simulink model "chaodianRM"  (R2021b)
settings: Solver=ode45  StartTime=0.0  StopTime=2  RelTol=1e-3  EnableMultiTasking=on
libraries: spsSeriesRLCBranchLib x9, spsCurrentMeasurementLib x4, spsMeanLib x2, simulink x2, spsVoltageMeasurementLib x2, spsDCVoltageSourceLib x1, spsMosfetLib x1, spsUniversalBridgeLib x1, spspowerguiLib x1
settings Model: SimulationMode=accelerator  Creator=bzz  LastModifiedBy=abc6820292
settings SolverCC: ZeroCrossAlgorithm=Adaptive  AlgebraicLoopSolver=TrustRegion
settings DataIOCC: LimitDataPoints=on  ReturnWorkspaceOutputs=off
settings OptimizationCC: LifeSpan=inf
settings DebuggingCC: AlgebraicLoopMsg=none  IgnoredZcDiagnostic=none  AllowSymbolicDim=off  SFUnexpectedBacktrackingDiag=warning  SFNoUnconditionalDefaultTransitionDiag=warning  SFMachineParentedDataDiag=warning  ArithmeticOperatorsInVariantConditions=warning
settings ModelReferenceCC: PropagateSignalLabelsOutOfModel=off
settings SFSimCC: SimUseLocalCustomCode=off  CustomCodeUndefinedFunction=UseInterfaceOnly
settings RTWCC: RTWUseLocalCustomCode=off
settings CodeAppCC: StateflowObjectComments=on
settings GRTTargetCC: TargetLangStandard=C89/C90 (ANSI)
settings ConfigComp: CovMetricSettings=dw  CovSaveCumulativeToWorkspaceVar=on  CovSaveSingleToWorkspaceVar=on  CovExternalEMLEnable=off
settings SimscapeCC: SimscapeNormalizeSystem=off

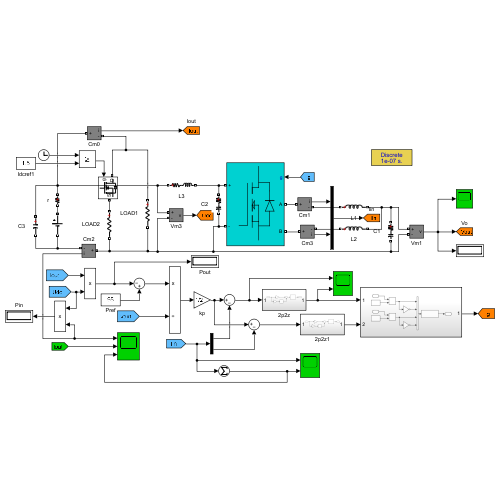
[thumbnail: Simulink's stored preview of the top-level diagram]
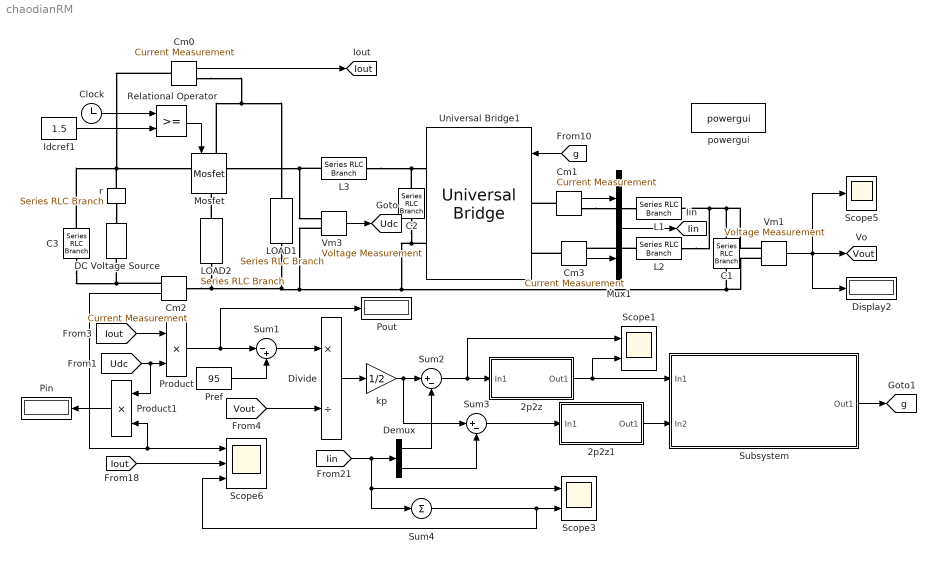
== system chaodianRM ==
  2p2z : Subsystem
  2p2z1 : Subsystem
  C1 : spsSeriesRLCBranchLib/Series RLC Branch  LConnTagsString=__new0  RConnTagsString=__new0  BranchType=RC  Resistance=0.05  Inductance=0  SetiL0=off  InitialCurrent=0  Capacitance=3.33  Setx0=on  InitialVoltage=20  Measurements=None
  C2 : spsSeriesRLCBranchLib/Series RLC Branch  LConnTagsString=__new0  RConnTagsString=__new0  BranchType=RC  Resistance=0.01  Inductance=0  SetiL0=off  InitialCurrent=0  Capacitance=10e-6  Setx0=on  InitialVoltage=24  Measurements=None
  C3 : spsSeriesRLCBranchLib/Series RLC Branch  LConnTagsString=__new0  RConnTagsString=__new0  BranchType=C  Resistance=0.01  Inductance=0  SetiL0=off  InitialCurrent=0  Capacitance=1e-3  Setx0=on  InitialVoltage=24  Measurements=None
  Clock : Clock
  Cm{0..3} (4 alike) : spsCurrentMeasurementLib/Current Measurement  PhasorSimulation=off  OutputType=Complex  PSBequivalent=0
  DC Voltage Source : spsDCVoltageSourceLib/DC Voltage Source  Amplitude=24  Measurements=None
  Demux : Demux  Outputs=2
  Display2 : Display
  Divide : Product  Inputs=*/
  Idcref1 : Constant  Value=1.5
  L1 : spsSeriesRLCBranchLib/Series RLC Branch  LConnTagsString=__new0  RConnTagsString=__new0  BranchType=L  Resistance=0  Inductance=2e-4  SetiL0=off  InitialCurrent=0  Capacitance=inf  Setx0=off  InitialVoltage=0  Measurements=None
  L2 : spsSeriesRLCBranchLib/Series RLC Branch  LConnTagsString=__new0  RConnTagsString=__new0  BranchType=L  Resistance=0  Inductance=2e-4  SetiL0=off  InitialCurrent=0  Capacitance=inf  Setx0=off  InitialVoltage=0  Measurements=None
  L3 : spsSeriesRLCBranchLib/Series RLC Branch  LConnTagsString=__new0  RConnTagsString=__new0  BranchType=RL  Resistance=0.05  Inductance=1e-5  SetiL0=off  InitialCurrent=0  Capacitance=inf  Setx0=off  InitialVoltage=0  Measurements=None
  LOAD1 : spsSeriesRLCBranchLib/Series RLC Branch  LConnTagsString=__new0  RConnTagsString=__new0  BranchType=R  Resistance=24  Inductance=2e-3  SetiL0=off  InitialCurrent=0  Capacitance=inf  Setx0=off  InitialVoltage=0  Measurements=None
  LOAD2 : spsSeriesRLCBranchLib/Series RLC Branch  LConnTagsString=__new0  RConnTagsString=__new0  BranchType=R  Resistance=6  Inductance=2e-3  SetiL0=off  InitialCurrent=0  Capacitance=inf  Setx0=off  InitialVoltage=0  Measurements=None
  Mosfet : spsMosfetLib/Mosfet  Ron=0.1  Lon=0  Rd=0.01  Vfd=0  IC=0  Rs=1e5  Cs=inf  Measurements=off
  Mux1 : Mux  Inputs=2
  Pin : Display
  Pout : Display
  Pref : Constant  Value=95
  Product : Product
  Product1 : Product
  Relational Operator : RelationalOperator  OutDataTypeStr=boolean  RndMeth=Nearest
  Scope1 : Scope  NumInputPorts=2
  Scope3 : Scope  NumInputPorts=2
  Scope5 : Scope
  Scope6 : Scope  NumInputPorts=3
  Subsystem : Subsystem
  Sum1 : Sum  Inputs=|-+
  Sum2 : Sum  Inputs=|+-
  Sum3 : Sum  Inputs=|+-
  Sum4 : Sum  Inputs=+
  Universal Bridge1 : spsUniversalBridgeLib/Universal Bridge  Arms=2  SnubberResistance=1e5  SnubberCapacitance=1e-9  Device=MOSFET / Diodes  Ron=1e-3  Lon=0  ForwardVoltages="[  0  0  ]"  ForwardVoltage=0  GTOparameters=[ 10e-6 , 20e-6 ]  IGBTparameters=[ 1e-6 , 2e-6 ]  Measurements=None  Measurements_2=None  converterType=Rectifier
  Vm1 : spsVoltageMeasurementLib/Voltage Measurement  PhasorSimulation=off  OutputType=Complex  PSBequivalent=0
  Vm3 : spsVoltageMeasurementLib/Voltage Measurement  PhasorSimulation=off  OutputType=Complex  PSBequivalent=0
  kp : Gain  Gain=1/2
  powergui : spspowerguiLib/powergui  SimulationMode=Discrete  SampleTime=1e-7  frequency=60  Iterations=50  frequencyindice=0  Pbase=100e6  ErrMax=1e-4  UnitsV=kV  UnitsW=MW  buscounter=0  FunctionMessages=off  echomessages=off  EnableUseOfTLC=off  CurrentSourceSwitches=off  DisableSnubberDevices=off  DisableRonSwitches=off  DisableVfSwitches=off  DisplayEquations=off  AutomaticDiscreteSolvers=off  SolverType=Tustin/Backward Euler (TBE)  Interpol=off  ExternalGateDelay=off  methode=off  Ts=0  x0status=blocks  SPID=off  SwTol=0  HookPort=off  NonlinearTolerance=1e-4  nMaxIteration=100  ContinueOnMaxIteration=off  RestoreLinks=warning  ResistiveCurrentMeasurement=off  Frange=[0:2:500]  Ylog=off  Xlog=on  ShowGrid=off  save=off  variable=ZData  structure=QQQQQ  ZoomFFT=off  StartTime=0.5  cycles=15  DisplayStyle=1  fundamental=50  FreqAxis=off  MaxFrequency=1000  frequencyindicesteady=1  RmsSteady=1  display=off
  r : spsSeriesRLCBranchLib/Series RLC Branch  LConnTagsString=__new0  RConnTagsString=__new0  BranchType=R  Resistance=0.05  Inductance=2e-3  SetiL0=off  InitialCurrent=0  Capacitance=inf  Setx0=off  InitialVoltage=0  Measurements=None
  tag scope: Iin=global, Iout=global, Udc=global, Vout=global, g=global
  wires:
  Vm3/1 -> [Udc]
  Vm1/1 -> Display2/1, Scope5/1, [Vout]
  [g] -> Universal Bridge1/1
  Cm0/1 -> [Iout]
  Cm2/1 -> Product1/2, Scope6/1
  Subsystem/1(Out1) -> [g]
  [Vout] -> Divide/2
  Cm3/1 -> Mux1/2
  Cm1/1 -> Mux1/1
  Mux1/1 -> [Iin]
  [Iin] -> Sum4/1, Scope3/1, Demux/1
  [Iout] -> Scope6/2
  Relational Operator/1 -> Mosfet/1
  Idcref1/1 -> Relational Operator/2
  Clock/1 -> Relational Operator/1
  Demux/1 -> Sum2/2
  Demux/2 -> Sum3/2
  Sum2/1 -> 2p2z/1(In1), Scope1/1
  Sum4/1 -> Scope6/3, Scope3/2
  2p2z/1(Out1) -> Scope1/2, Subsystem/1(In1)
  2p2z1/1(Out1) -> Subsystem/2(In2)
  Sum3/1 -> 2p2z1/1(In1)
  [Iout] -> Product/1
  [Udc] -> Product1/1, Product/2
  Product/1 -> Pout/1, Sum1/1
  Sum1/1 -> Divide/1
  Pref/1 -> Sum1/2
  Divide/1 -> kp/1
  kp/1 -> Sum3/1, Sum2/1
  Product1/1 -> Pin/1
  connections:
  Cm0/LConn1 -- C3/LConn1 -- r/LConn1 -- L3/LConn1 -- Vm3/LConn1
  C1/LConn1 -- Vm1/LConn1 -- L2/RConn1 -- L1/RConn1
  Cm1/LConn1 -- Universal Bridge1/LConn1
  Cm1/RConn1 -- L1/LConn1
  Vm1/LConn2 -- C2/RConn1 -- Universal Bridge1/RConn2 -- LOAD2/RConn1 -- Cm2/LConn1 -- LOAD1/RConn1 -- Vm3/LConn2 -- C1/RConn1
  Cm0/RConn1 -- Mosfet/LConn1 -- LOAD1/LConn1
  Cm2/RConn1 -- C3/RConn1 -- DC Voltage Source/LConn1
  Cm3/LConn1 -- Universal Bridge1/LConn2
  L2/LConn1 -- Cm3/RConn1
  LOAD2/LConn1 -- Mosfet/RConn1
  L3/RConn1 -- C2/LConn1 -- Universal Bridge1/RConn1
  r/RConn1 -- DC Voltage Source/RConn1

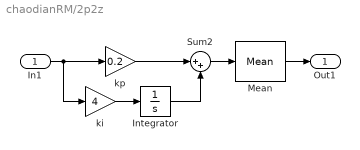
== system chaodianRM/2p2z ==
  In1 : Inport
  Integrator : Integrator  LimitOutput=on  UpperSaturationLimit=0.98  LowerSaturationLimit=0
  Mean : spsMeanLib/Mean  Freq=10000  Vinit=0  Ts=0
  Sum2 : Sum  Inputs=|++
  ki : Gain  Gain=4
  kp : Gain  Gain=0.2
  Out1 : Outport
  wires:
  In1/1 -> ki/1, kp/1
  ki/1 -> Integrator/1
  kp/1 -> Sum2/1
  Integrator/1 -> Sum2/2
  Sum2/1 -> Mean/1
  Mean/1 -> Out1/1

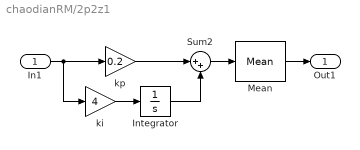
== system chaodianRM/2p2z1 ==
  In1 : Inport
  Integrator : Integrator  LimitOutput=on  UpperSaturationLimit=0.98  LowerSaturationLimit=0
  Mean : spsMeanLib/Mean  Freq=10000  Vinit=0  Ts=0
  Sum2 : Sum  Inputs=|++
  ki : Gain  Gain=4
  kp : Gain  Gain=0.2
  Out1 : Outport
  wires:
  In1/1 -> ki/1, kp/1
  ki/1 -> Integrator/1
  kp/1 -> Sum2/1
  Integrator/1 -> Sum2/2
  Sum2/1 -> Mean/1
  Mean/1 -> Out1/1

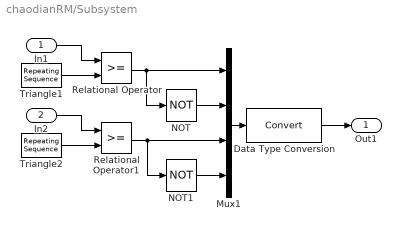
== system chaodianRM/Subsystem ==
  In1 : Inport
  In2 : Inport  Port=2
  Data Type Conversion : DataTypeConversion
  Mux1 : Mux
  NOT : Logic  Operator=NOT  IconShape=distinctive  AllPortsSameDT=off  OutDataTypeStr=boolean
  NOT1 : Logic  Operator=NOT  IconShape=distinctive  AllPortsSameDT=off  OutDataTypeStr=boolean
  Relational Operator : RelationalOperator  OutDataTypeStr=boolean  RndMeth=Nearest
  Relational Operator1 : RelationalOperator  OutDataTypeStr=boolean  RndMeth=Nearest
  Triangle1 : simulink/Sources/Repeating Sequence  rep_seq_t=[0 1/40000/2 1/40000]  rep_seq_y=[0 1 0]
  Triangle2 : simulink/Sources/Repeating Sequence  rep_seq_t=[0 1/40000/2 1/40000]  rep_seq_y=[1 0 1]
  Out1 : Outport
  wires:
  Relational Operator/1 -> NOT/1, Mux1/1
  Triangle2/1 -> Relational Operator1/2
  Relational Operator1/1 -> NOT1/1, Mux1/3
  Data Type Conversion/1 -> Out1/1
  Mux1/1 -> Data Type Conversion/1
  Triangle1/1 -> Relational Operator/2
  NOT1/1 -> Mux1/4
  In2/1 -> Relational Operator1/1
  NOT/1 -> Mux1/2
  In1/1 -> Relational Operator/1
